simulink library "did"  (R2021b)
settings: Solver=VariableStepAuto  StartTime=0.0  StopTime=10.0  RelTol=1e-3
undefined symbols (not defined in the file or in its folder): ADID_DODRange_pct, ADID_SOCRange_pct, ADID_TempRange_C, DiscIntNeverNeededParam, ENUM_CHRGPLUGSTA_AC, ENUM_CHRGPLUGSTA_DC, ENUM_CHRGPLUGSTA_NONE, ENUM_DRIVETRAIN_AWD, ENUM_DRIVETRAIN_FWD, ENUM_DRIVETRAIN_RWD, ENUM_EXTCHRGSTS_CHARGING, ENUM_OBCV2LSTA_WORKING, ENUM_PWRSTASW_READY, ENUM_VEHICLETYPE_D31HAWD, ENUM_VEHICLETYPE_D31HRWD, HOUR2SEC, HUNDRED, KDID_CPSAVehSpdThres_kph, KDID_DIDModelVersion_raw, KDID_DoDChrgCycle_s, KDID_FiveKmEquivEnergy_Wh, KDID_FlashInitDIDModelVersion_raw, KDID_IPSAVehSpdThres_kph, KDID_PropActiveTripThres_s, KDID_PSARResetThres_sec, KDID_RESSCNTSDODRNGAXIS_enum, KDID_RESSTIMESOCRNGAXIS_enum, KDID_RESSTTEMPRNGAXIS_enum, KDID_WarnUpPropActiveThres_s, KDID_WarnUpVehOperIdleThres_mph, KDID_WarnUpVehOperIdleThres_s, KDID_WarnUpVehOperThres_mph, KDID_WarnUpVehOperThres_s, KPH2MPH, KXX2XX, MINUSONE_FLOAT, ONE_FLOAT, ONE_INT, ONE_INT16, ONE_PERCENT, TRUE, UINT16_MAX, UINT32_MAX, XX2KXX, ZERO_FLOAT, ZERO_INT, ZERO_INT16, ZERO_INT32
libraries: hcu_lib x112, simulink x10, nmm x1
(part 1 of 4)
settings Model: Creator=FVT23010  LastModifiedBy=FVT23010

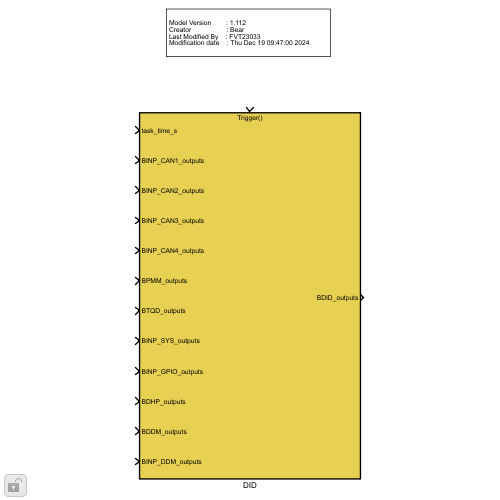
[thumbnail: Simulink's stored preview of the top-level diagram]
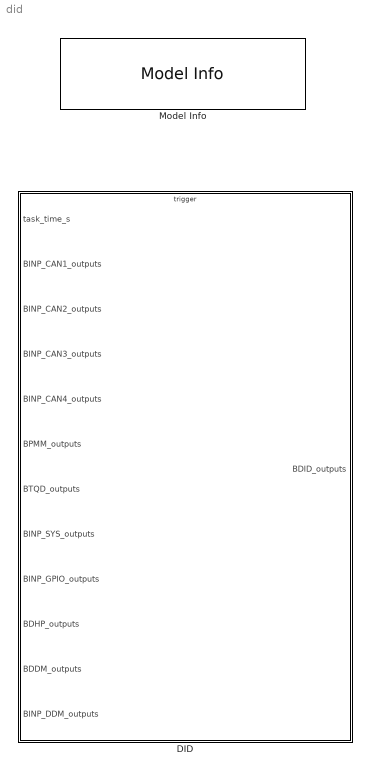
== system did ==
  DID : Subsystem
      settings: RTWSystemCode=Nonreusable function  RTWFcnNameOpts=Use subsystem name  RTWFileNameOpts=Use subsystem name
  Model Info : nmm/Model Info  InitialBlockCM=None  BlockCM=None  Frame=on  DisplayStringWithTags=|  HorizontalTextAlignment=Left  LeftAlignmentValue=0.02  SourceBlockDiagram=pmm  TagMaxNumber=20
      | Model Version        : %<ModelVersion>
      | Creator                   : Bear
      | Last Modified By    : %<LastModifiedBy>
      | Modification date    : %<LastModificationDate>

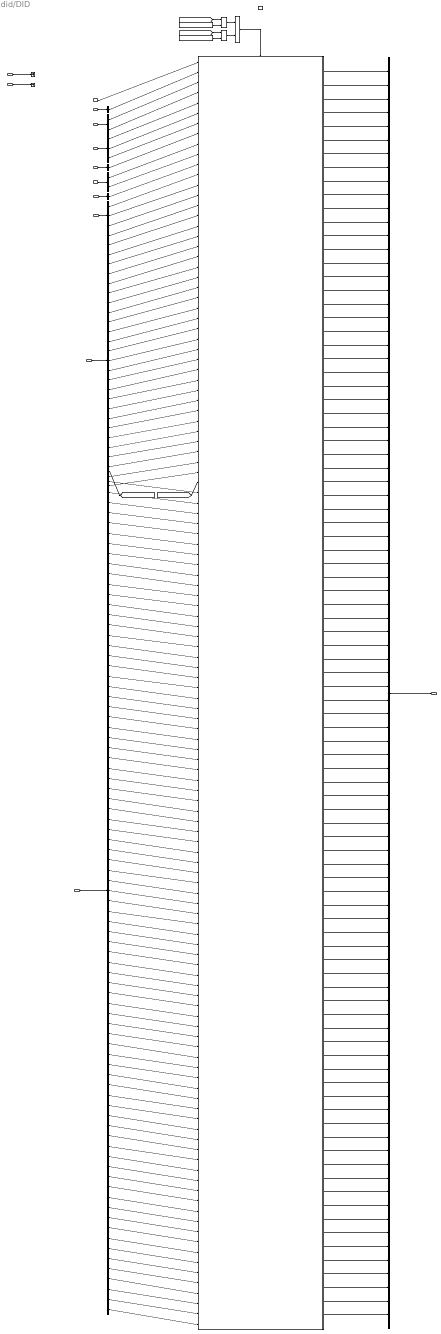
== system did/DID ==
  task_time_s : Inport
  BINP_CAN1_outputs : Inport  Port=2  OutDataTypeStr=Bus: BINP_CAN1_outputs
  BINP_CAN2_outputs : Inport  Port=3  OutDataTypeStr=Bus: BINP_CAN2_outputs
  BINP_CAN3_outputs : Inport  Port=4  OutDataTypeStr=Bus: BINP_CAN3_outputs
  BINP_CAN4_outputs : Inport  Port=5  OutDataTypeStr=Bus: BINP_CAN4_outputs
  BPMM_outputs : Inport  Port=6  OutDataTypeStr=Bus: BPMM_outputs
  BTQD_outputs : Inport  Port=7  OutDataTypeStr=Bus: BTQD_outputs
  BINP_SYS_outputs : Inport  Port=8  OutDataTypeStr=Bus: BINP_SYS_outputs
  BINP_GPIO_outputs : Inport  Port=9  OutDataTypeStr=Bus: BINP_GPIO_outputs
  BDHP_outputs : Inport  Port=10  OutDataTypeStr=Bus: BDHP_outputs
  BDDM_outputs : Inport  Port=11  OutDataTypeStr=Bus: BDDM_outputs
  BINP_DDM_outputs : Inport  Port=12  OutDataTypeStr=Bus: BINP_DDM_outputs
  Trigger : TriggerPort  TriggerType=function-call  VariantControl=(inherit)  PortDimensions=1
  Bus Creator : BusCreator  Inputs=92  OutDataTypeStr=Bus: BDID_outputs  NonVirtualBus=on
  Bus Selector : BusSelector  OutputSignals=VINP_VehicleType_enum,VINP_CarModel1_cnt,VINP_CarModel2_cnt,VINP_CarModel3_cnt,VINP_ECU1_cnt,VINP_ECU2_cnt,VINP_Major1_cnt,VINP_Major2_cnt,VINP_Minor1_cnt,VINP_Minor2_cnt,VINP_Patch1_cnt,VINP_Patch2_cnt,VINP_Country1_cnt,VINP_Country2_cnt,VINP_Variation_cnt,VINP_ECUGen1_cnt,VINP_ECUGen2_cnt,VINP_FlashMILDIST_km,VINP_FlashWARMUPS_cnt,VINP_FlashCLRDIST_km,VINP_FlashMILTIME_min,VINP_FlashCLRTIME_min,VINP_FlashNUMPSATRIPSFLTMEMCLR_cnt,VINP_FlashPSAR_sec,VINP_FlashPSAL_sec,VINP_FlashIPSAR_sec,VINP_FlashIPSAL_sec,VINP_FlashCPSAR_sec,VINP_FlashCPSAL_sec,VINP_FlashHVBNAH_Ahr,VINP_FlashIGNCNTR_cnt,VINP_FlashTNBCPSAR_Ahr,VINP_FlashTNBCPSAL_Ahr,VINP_FlashTNECPSAR_kWh,VINP_FlashTNECPSAL_kWh,VINP_FlashTEBPSAR_kWh,VINP_FlashTEBPSAL_kWh,VINP_FlashTGEOVCR_kWh,VINP_FlashTGEOVCL_kWh,VINP_FlashGECHGOVCDCR_kWh,VINP_FlashGECHGOVCDCL_kWh,VINP_FlashGECHGOVCACR_kWh,VINP_FlashGECHGOVCACL_kWh,VINP_FlashRESSV2XENNONPSAR_kWh,VINP_FlashRESSV2XENNONPSAL_kWh,VINP_FlashODOMETER_km,VINP_FlashPKERNumerator_kphsqr,VINP_FlashPKELNumerator_kphsqr,VINP_FlashResetCDEODTR_km,VINP_FlashBattTempPSAR_sec,VINP_FlashAvgBattTempPSAR_C,VINP_FlashBattTempPSAL_sec,VINP_FlashAvgBattTempPSAL_C,VINP_FlashOVCR_sec,VINP_FlashAvgBattTempOVCR_C,VINP_FlashOVCL_sec,VINP_FlashAvgBattTempOVCL_C,VINP_FlashOFFR_sec,VINP_FlashAvgBattTempOFFR_C,VINP_FlashOFFL_sec,VINP_FlashAvgBattTempOFFL_C,VINP_FlashHVBNE_kWh,VINP_FlashQTYPSATRIPSR_cnt,VINP_FlashQTYPSATRIPSL_cnt,VINP_FlashRESSCNTDODRNGR_cnt,VINP_FlashETMBTOER_kWh,VINP_FlashETMBTOEL_kWh,VINP_FlashRESSCNTDODRNGL_cnt,VINP_FlashETMATOER_kWh,VINP_FlashETMATOEL_kWh,VINP_FlashRESSTIMESOCPSARNGR_s,VINP_FlashRESSTIMESOCPSARNGL_s,VINP_FlashRESSTIMESOCCHGRNGR_s,VINP_FlashRESSTIMESOCOFFRNGL_s,VINP_FlashMAXBATTEMPL_C,VINP_FlashMINBATTEMPL_C,VINP_FlashRESSTIMESOCCHGRNGL_s,VINP_FlashRESSTIMESOCOFFRNGR_s,VINP_FlashAVGBATTEMPL_sec,VINP_FlashAVGBATTEMPL_C,VINP_VinCode_cnt,VINP_FlashDIDModelVersion_raw,VINP_FlashDIDModelVersionChkSum_raw
  Bus Selector1 : BusSelector  OutputSignals=VTQD_VehActSpd_kph
  Bus Selector2 : BusSelector  OutputSignals=VPMM_SysPowerMode_enum,VPMM_DrivetrainSelect_enum
  Bus Selector3 : BusSelector  OutputSignals=VDDM_VehMalfunLevel_enum,VDDM_LimpHomeActTmp_flg,VDDM_EnterNewOperCyc_flg
  Bus Selector4 : BusSelector  OutputSignals=VINP_ODOMETER_km,VINP_CANMsgValidMETER1_flg
  Bus Selector5 : BusSelector  OutputSignals=VINP_HVBattSOC_pct,VINP_HVBattPackVolt_V,VINP_ExtChrgSta_enum,VINP_HVBattCurr_A,VINP_HVBattVolt_V,VINP_ChrgPlugSta_enum,VINP_HVBPwrAvailChrg_kW,VINP_HVBCellVoltMax_mV,VINP_HVBCellVoltMin_mV,VINP_HVBSOH_pct,VINP_CANMsgValidMCUBR1_flg,VINP_CANMsgValidBMS6_flg,VINP_CANMsgValidBMS1_flg,VINP_CANMsgValidCCU2_flg,VINP_CANMsgValidBMS4_flg,VINP_CellTempAvg_C,VINP_OBCV2LSta_enum,VINP_RrMCUDCBusCurr_A,VINP_RrMCUDCBusVolt_V,VINP_FrMCUDCBusCurr_A,VINP_FrMCUDCBusVolt_V,VINP_CANMsgValidMCUBF1_flg,VINP_HVBMTempMax_C,VINP_HVBMTempMin_C,VINP_MCUBRRealPwrKwSta_kW,VINP_MCUBFRealPwrKwSta_kW,VINP_CANMsgValidBMS3_flg
  Bus Selector6 : BusSelector  OutputSignals=VINP_ClearDTCcmd_flg
  Bus Selector7 : BusSelector  OutputSignals=VDHP_LowIdleAccPedal_flg,VDHP_EAPS1NRM_pct,VDHP_EAPS2NRM_pct
  Bus Selector8 : BusSelector  OutputSignals=VINP_CANMsgValidESC1_flg
  Constant : Constant  Value=ENUM_VEHICLETYPE_D31HAWD
  Constant1 : Constant  Value=ENUM_VEHICLETYPE_D31HRWD
  Equal : RelationalOperator  Operator===  OutDataTypeStr=boolean  RndMeth=Simplest
  Equal1 : RelationalOperator  Operator===  OutDataTypeStr=boolean  RndMeth=Simplest
  Logical Operator : Logic  Operator=OR  AllPortsSameDT=off  OutDataTypeStr=boolean
  Subsystem : Subsystem
  Terminator : Terminator
  Terminator1 : Terminator
  BDID_outputs : Outport  OutDataTypeStr=Bus: BDID_outputs
  wires:
  BTQD_outputs/1 -> Bus Selector1/1
  task_time_s/1 -> Subsystem/1(task_time_s)
  Bus Selector1/1 -> Subsystem/2(VTQD_VehActSpd_kph)  "<VTQD_VehActSpd_kph>"
  BPMM_outputs/1 -> Bus Selector2/1
  Bus Selector2/1 -> Subsystem/3(VPMM_SysPowerMode_enum)  "<VPMM_SysPowerMode_enum>"
  BDDM_outputs/1 -> Bus Selector3/1
  BINP_CAN2_outputs/1 -> Bus Selector4/1
  Bus Selector3/1 -> Subsystem/5(VDDM_VehMalfunLevel_enum)  "<VDDM_VehMalfunLevel_enum>"
  Bus Selector4/1 -> Subsystem/9(VINP_ODOMETER_km)  "<VINP_ODOMETER_km>"
  BINP_DDM_outputs/1 -> Bus Selector6/1
  Bus Selector6/1 -> Subsystem/11(VINP_ClearDTCcmd_flg)  "<VINP_ClearDTCcmd_flg>"
  Bus Selector4/2 -> Subsystem/10(VINP_CANMsgValidMETER1_flg)  "<VINP_CANMsgValidMETER1_flg>"
  Bus Selector3/2 -> Subsystem/6(VDDM_LimpHomeActTmp_flg)  "<VDDM_LimpHomeActTmp_flg>"
  Bus Selector3/3 -> Subsystem/7(VDDM_EnterNewOperCyc_flg)  "<VDDM_EnterNewOperCyc_flg>"
  BDHP_outputs/1 -> Bus Selector7/1
  Bus Selector7/1 -> Subsystem/12(VDHP_LowIdleAccPedal_flg)  "<VDHP_LowIdleAccPedal_flg>"
  Bus Selector7/2 -> Subsystem/13(VDHP_EAPS1NRM_pct)  "<VDHP_EAPS1NRM_pct>"
  Bus Selector7/3 -> Subsystem/14(VDHP_EAPS2NRM_pct)  "<VDHP_EAPS2NRM_pct>"
  Bus Selector5/1 -> Subsystem/15(VINP_HVBattSOC_pct)  "<VINP_HVBattSOC_pct>"
  Bus Selector5/2 -> Subsystem/16(VINP_HVBattPackVolt_V)  "<VINP_HVBattPackVolt_V>"
  Constant/1 -> Equal/2
  Constant1/1 -> Equal1/2
  Equal/1 -> Logical Operator/1
  Equal1/1 -> Logical Operator/2
  Logical Operator/1 -> Subsystem/Enable
  Bus Selector5/3 -> Subsystem/17(VINP_ExtChrgSta_enum)  "<VINP_ExtChrgSta_enum>"
  BINP_CAN3_outputs/1 -> Bus Selector5/1
  Bus Selector5/4 -> Subsystem/18(VINP_HVBattCurr_A)  "<VINP_HVBattCurr_A>"
  Bus Selector5/5 -> Subsystem/19(VINP_HVBattVolt_V)  "<VINP_HVBattVolt_V>"
  Bus Selector5/6 -> Subsystem/20(VINP_ChrgPlugSta_enum)  "<VINP_ChrgPlugSta_enum>"
  Bus Selector5/7 -> Subsystem/21(VINP_HVBPwrAvailChrg_kW)  "<VINP_HVBPwrAvailChrg_kW>"
  Bus Selector5/8 -> Subsystem/22(VINP_HVBCellVoltMax_mV)  "<VINP_HVBCellVoltMax_mV>"
  Bus Selector5/9 -> Subsystem/23(VINP_HVBCellVoltMin_mV)  "<VINP_HVBCellVoltMin_mV>"
  Bus Selector5/10 -> Subsystem/24(VINP_HVBSOH_pct)  "<VINP_HVBSOH_pct>"
  BINP_CAN1_outputs/1 -> Bus Selector8/1  "BINP_CAN1_outputs"
  Bus Selector5/11 -> Subsystem/25(VINP_CANMsgValidMCUBR1_flg)  "<VINP_CANMsgValidMCUBR1_flg>"
  Bus Selector8/1 -> Subsystem/8(VINP_CANMsgValidESC1_flg)  "<VINP_CANMsgValidESC1_flg>"
  BINP_CAN4_outputs/1 -> Terminator/1
  BINP_GPIO_outputs/1 -> Terminator1/1
  Subsystem/4(VDID_WARMUPS_cnt) -> Bus Creator/4
  Subsystem/5(VDID_CLRDIST_km) -> Bus Creator/5
  Subsystem/3(VDID_MILDIST_km) -> Bus Creator/3
  Subsystem/6(VDID_APPD_pct) -> Bus Creator/6
  Subsystem/2(VDID_RUNTM_s) -> Bus Creator/2
  Subsystem/7(VDID_APPE_pct) -> Bus Creator/7
  Subsystem/1(VDID_VSS_kph) -> Bus Creator/1
  Subsystem/8(VDID_MILTIME_min) -> Bus Creator/8
  Subsystem/9(VDID_CLRTIME_min) -> Bus Creator/9
  Subsystem/10(VDID_BATSOC_pct) -> Bus Creator/10
  Subsystem/11(VDID_HEVBATT_V) -> Bus Creator/11
  Subsystem/12(VDID_ODOMETER_km) -> Bus Creator/12
  Subsystem/13(VDID_BATSOH_pct) -> Bus Creator/13
  Subsystem/14(VDID_HVBCellVoltMin_V) -> Bus Creator/14
  Subsystem/15(VDID_HVBCellVoltMax_V) -> Bus Creator/15
  Subsystem/16(VDID_HVESSCHARGELIM_kW) -> Bus Creator/16
  Subsystem/17(VDID_HVESSCHARGEACT_kW) -> Bus Creator/17
  Subsystem/18(VDID_HVESSENER_Whps) -> Bus Creator/18
  Subsystem/19(VDID_NUMPSATRIPSFLTMEMCLR_cnt) -> Bus Creator/19
  Subsystem/20(VDID_HVBattCurr_Ahps) -> Bus Creator/20
  Subsystem/21(VDID_PSAR_sec) -> Bus Creator/21
  Subsystem/22(VDID_PSAL_sec) -> Bus Creator/22
  Subsystem/23(VDID_IPSAR_sec) -> Bus Creator/23
  Subsystem/24(VDID_IPSAL_sec) -> Bus Creator/24
  Subsystem/25(VDID_CPSAR_sec) -> Bus Creator/25
  Subsystem/26(VDID_CPSAL_sec) -> Bus Creator/26
  Subsystem/27(VDID_HVBNAH_Ahr) -> Bus Creator/27
  Subsystem/28(VDID_HVBNE_kWh) -> Bus Creator/28
  Subsystem/29(VDID_IGNCNTR_cnt) -> Bus Creator/29
  Subsystem/30(VDID_TNBCPSAR_Ahr) -> Bus Creator/30
  Subsystem/31(VDID_TNBCPSAL_Ahr) -> Bus Creator/31
  Subsystem/32(VDID_TNECPSAR_kWh) -> Bus Creator/32
  Subsystem/33(VDID_TNECPSAL_kWh) -> Bus Creator/33
  Subsystem/34(VDID_TEBPSAR_kWh) -> Bus Creator/34
  Subsystem/35(VDID_TEBPSAL_kWh) -> Bus Creator/35
  Subsystem/36(VDID_TGEOVCR_kWh) -> Bus Creator/36
  Subsystem/37(VDID_TGEOVCL_kWh) -> Bus Creator/37
  Subsystem/38(VDID_GECHGOVCDCR_kWh) -> Bus Creator/38
  Subsystem/39(VDID_GECHGOVCDCL_kWh) -> Bus Creator/39
  Subsystem/40(VDID_GECHGOVCACR_kWh) -> Bus Creator/40
  Subsystem/41(VDID_GECHGOVCACL_kWh) -> Bus Creator/41
  Subsystem/42(VDID_RESSV2XENNONPSAR_kWh) -> Bus Creator/42
  Subsystem/43(VDID_RESSV2XENNONPSAL_kWh) -> Bus Creator/43
  Subsystem/44(VDID_PKER_kphsqr) -> Bus Creator/44
  Subsystem/45(VDID_PKEL_kphsqr) -> Bus Creator/45
  Subsystem/46(VDID_ResetCDEODTR_km) -> Bus Creator/46
  Subsystem/47(VDID_CDEODTR_km) -> Bus Creator/47
  Subsystem/48(VDID_CDEODTL_km) -> Bus Creator/48
  Subsystem/49(VDID_AvgBattTempPSAR_C) -> Bus Creator/49
  Subsystem/50(VDID_AvgBattTempPSAL_C) -> Bus Creator/50
  Subsystem/51(VDID_AvgBattTempOVCR_C) -> Bus Creator/51
  Subsystem/52(VDID_AvgBattTempOVCL_C) -> Bus Creator/52
  Subsystem/53(VDID_AvgBattTempOFFR_C) -> Bus Creator/53
  Subsystem/54(VDID_AvgBattTempOFFL_C) -> Bus Creator/54
  Bus Creator/1 -> BDID_outputs/1
  Bus Selector5/12 -> Subsystem/26(VINP_CANMsgValidBMS6_flg)  "<VINP_CANMsgValidBMS6_flg>"
  Bus Selector5/13 -> Subsystem/27(VINP_CANMsgValidBMS1_flg)  "<VINP_CANMsgValidBMS1_flg>"
  Bus Selector5/14 -> Subsystem/28(VINP_CANMsgValidCCU2_flg)  "<VINP_CANMsgValidCCU2_flg>"
  Bus Selector5/15 -> Subsystem/29(VINP_CANMsgValidBMS4_flg)  "<VINP_CANMsgValidBMS4_flg>"
  Bus Selector5/16 -> Subsystem/30(VINP_CellTempAvg_C)  "<VINP_CellTempAvg_C>"
  Bus Selector5/17 -> Subsystem/31(VINP_OBCV2LSta_enum)  "<VINP_OBCV2LSta_enum>"
  Subsystem/55(VDID_QTYPSATRIPSR_cnt) -> Bus Creator/55
  Subsystem/56(VDID_QTYPSATRIPSL_cnt) -> Bus Creator/56
  Subsystem/57(VDID_RESSCNTDODRNGR_cnt) -> Bus Creator/57
  Subsystem/58(VDID_RESSCNTDODRNGL_cnt) -> Bus Creator/58
  Subsystem/59(VDID_ETMATOER_kWh) -> Bus Creator/59
  Subsystem/60(VDID_ETMATOEL_kWh) -> Bus Creator/60
  Subsystem/61(VDID_ETMBTOER_kWh) -> Bus Creator/61
  Subsystem/62(VDID_ETMBTOEL_kWh) -> Bus Creator/62
  Subsystem/63(VDID_RESSTIMESOCPSARNGR_s) -> Bus Creator/63
  Subsystem/64(VDID_RESSTIMESOCPSARNGL_s) -> Bus Creator/64
  Subsystem/65(VDID_RESSTIMESOCCHGRNGR_s) -> Bus Creator/65
  Subsystem/66(VDID_RESSTIMESOCCHGRNGL_s) -> Bus Creator/66
  Subsystem/67(VDID_RESSTIMESOCOFFRNGR_s) -> Bus Creator/67
  Subsystem/68(VDID_RESSTIMESOCOFFRNGL_s) -> Bus Creator/68
  Subsystem/69(VDID_MAXBATTEMPL_C) -> Bus Creator/69
  Subsystem/70(VDID_MINBATTEMPL_C) -> Bus Creator/70
  Subsystem/71(VDID_AVGBATTEMPL_C) -> Bus Creator/71
  Subsystem/72(VDID_PRO TOCOLID_enum) -> Bus Creator/72
  Bus Selector5/24 -> Subsystem/38(VINP_HVBMTempMin_C)  "<VINP_HVBMTempMin_C>"
  Bus Selector5/23 -> Subsystem/37(VINP_HVBMTempMax_C)  "<VINP_HVBMTempMax_C>"
  Bus Selector5/22 -> Subsystem/36(VINP_CANMsgValidMCUBF1_flg)  "<VINP_CANMsgValidMCUBF1_flg>"
  Bus Selector5/21 -> Subsystem/35(VINP_FrMCUDCBusVolt_V)  "<VINP_FrMCUDCBusVolt_V>"
  Bus Selector5/20 -> Subsystem/34(VINP_FrMCUDCBusCurr_A)  "<VINP_FrMCUDCBusCurr_A>"
  Bus Selector5/19 -> Subsystem/33(VINP_RrMCUDCBusVolt_V)  "<VINP_RrMCUDCBusVolt_V>"
  Bus Selector5/18 -> Subsystem/32(VINP_RrMCUDCBusCurr_A)  "<VINP_RrMCUDCBusCurr_A>"
  Subsystem/73(VDID_RESSTTEMPRNGAXIS_enum) -> Bus Creator/73
  Subsystem/74(VDID_RESSTIMESOCRNGAXIS_enum) -> Bus Creator/74
  Subsystem/75(VDID_RESSCNTSDODRNGAXIS_enum) -> Bus Creator/75
  Bus Selector5/27 -> Subsystem/41(VINP_CANMsgValidBMS3_flg)  "<VINP_CANMsgValidBMS3_flg>"
  Bus Selector/2 -> Subsystem/43(VINP_CarModel1_cnt)  "<VINP_CarModel1_cnt>"
  Bus Selector/3 -> Subsystem/44(VINP_CarModel2_cnt)  "<VINP_CarModel2_cnt>"
  Bus Selector/4 -> Subsystem/45(VINP_CarModel3_cnt)  "<VINP_CarModel3_cnt>"
  Bus Selector/5 -> Subsystem/46(VINP_ECU1_cnt)  "<VINP_ECU1_cnt>"
  Bus Selector/6 -> Subsystem/47(VINP_ECU2_cnt)  "<VINP_ECU2_cnt>"
  Bus Selector/7 -> Subsystem/48(VINP_Major1_cnt)  "<VINP_Major1_cnt>"
  Bus Selector/8 -> Subsystem/49(VINP_Major2_cnt)  "<VINP_Major2_cnt>"
  Bus Selector/9 -> Subsystem/50(VINP_Minor1_cnt)  "<VINP_Minor1_cnt>"
  Bus Selector/10 -> Subsystem/51(VINP_Minor2_cnt)  "<VINP_Minor2_cnt>"
  Bus Selector/11 -> Subsystem/52(VINP_Patch1_cnt)  "<VINP_Patch1_cnt>"
  Bus Selector/12 -> Subsystem/53(VINP_Patch2_cnt)  "<VINP_Patch2_cnt>"
  Bus Selector/13 -> Subsystem/54(VINP_Country1_cnt)  "<VINP_Country1_cnt>"
  Bus Selector/14 -> Subsystem/55(VINP_Country2_cnt)  "<VINP_Country2_cnt>"
  Bus Selector/15 -> Subsystem/56(VINP_Variation_cnt)  "<VINP_Variation_cnt>"
  Bus Selector/16 -> Subsystem/57(VINP_ECUGen1_cnt)  "<VINP_ECUGen1_cnt>"
  Bus Selector/17 -> Subsystem/58(VINP_ECUGen2_cnt)  "<VINP_ECUGen2_cnt>"
  [VINP_VehicleType_enum] -> Equal/1
  [VINP_VehicleType_enum] -> Equal1/1
  Subsystem/76(VDID_CALID_cnt) -> Bus Creator/76
  Subsystem/77(VDID_ECUNAME_cnt) -> Bus Creator/77
  Subsystem/78(VDID_PKERNumerator_kphsqr) -> Bus Creator/78
  Subsystem/79(VDID_PKELNumerator_kphsqr) -> Bus Creator/79
  Subsystem/80(VDID_BattTempPSAR_sec) -> Bus Creator/80
  Subsystem/81(VDID_BattTempPSAL_sec) -> Bus Creator/81
  Subsystem/82(VDID_OVCR_sec) -> Bus Creator/82
  Subsystem/83(VDID_OVCL_sec) -> Bus Creator/83
  Subsystem/84(VDID_OFFR_sec) -> Bus Creator/84
  Subsystem/85(VDID_OFFL_sec) -> Bus Creator/85
  Subsystem/86(VDID_AVGBATTEMPL_sec) -> Bus Creator/86
  Bus Selector2/2 -> Subsystem/4(VPMM_DrivetrainSelect_enum)  "<VPMM_DrivetrainSelect_enum>"
  Bus Selector/18 -> Subsystem/59(VINP_FlashMILDIST_km)  "<VINP_FlashMILDIST_km>"
  Bus Selector/19 -> Subsystem/60(VINP_FlashWARMUPS_cnt)  "<VINP_FlashWARMUPS_cnt>"
  Bus Selector/20 -> Subsystem/61(VINP_FlashDelayCLRDIST_km)  "<VINP_FlashCLRDIST_km>"
  Bus Selector/21 -> Subsystem/62(VINP_FlashMILTime_min)  "<VINP_FlashMILTIME_min>"
  Bus Selector/22 -> Subsystem/63(VINP_FlashCLRTime_min)  "<VINP_FlashCLRTIME_min>"
  Bus Selector/23 -> Subsystem/64(VINP_FlashNUMPSATRIPSFLTMEMCLR_cnt)  "<VINP_FlashNUMPSATRIPSFLTMEMCLR_cnt>"
  Bus Selector/24 -> Subsystem/65(VINP_FlashPSAR_sec)  "<VINP_FlashPSAR_sec>"
  Bus Selector/25 -> Subsystem/66(VINP_FlashPSAL_sec)  "<VINP_FlashPSAL_sec>"
  Bus Selector/26 -> Subsystem/67(VINP_FlashIPSAR_sec)  "<VINP_FlashIPSAR_sec>"
  Bus Selector/27 -> Subsystem/68(VINP_FlashIPSAL_sec)  "<VINP_FlashIPSAL_sec>"
  Bus Selector/28 -> Subsystem/69(VINP_FlashCPSAR_sec)  "<VINP_FlashCPSAR_sec>"
  Bus Selector/29 -> Subsystem/70(VINP_FlashCPSAL_sec)  "<VINP_FlashCPSAL_sec>"
  Bus Selector/30 -> Subsystem/71(VINP_FlashHVBNAH_Ah)  "<VINP_FlashHVBNAH_Ahr>"
  Bus Selector/31 -> Subsystem/72(VINP_FlashIGNCNTR_cnt)  "<VINP_FlashIGNCNTR_cnt>"
  Bus Selector/32 -> Subsystem/73(VINP_FlashTNBCPSAR_Ahr)  "<VINP_FlashTNBCPSAR_Ahr>"
  Bus Selector/33 -> Subsystem/74(VINP_FlashTNBCPSAL_Ahr)  "<VINP_FlashTNBCPSAL_Ahr>"
  Bus Selector/34 -> Subsystem/75(VINP_FlashTNECPSAR_kWh)  "<VINP_FlashTNECPSAR_kWh>"
  Bus Selector/35 -> Subsystem/76(VINP_FlashTNECPSAL_kWh)  "<VINP_FlashTNECPSAL_kWh>"
  Bus Selector/36 -> Subsystem/77(VINP_FlashTEBPSAR_kWh)  "<VINP_FlashTEBPSAR_kWh>"
  Bus Selector/37 -> Subsystem/78(VINP_FlashTEBPSAL_kWh)  "<VINP_FlashTEBPSAL_kWh>"
  Bus Selector/38 -> Subsystem/79(VINP_FlashTGEOVCR_kWh)  "<VINP_FlashTGEOVCR_kWh>"
  Bus Selector/39 -> Subsystem/80(VINP_FlashTGEOVCL_kWh)  "<VINP_FlashTGEOVCL_kWh>"
  Bus Selector/40 -> Subsystem/81(VINP_FlashGECHGOVCDCR_kWh)  "<VINP_FlashGECHGOVCDCR_kWh>"
  Bus Selector/41 -> Subsystem/82(VINP_FlashGECHGOVCDCL_kWh)  "<VINP_FlashGECHGOVCDCL_kWh>"
  Bus Selector/42 -> Subsystem/83(VINP_FlashGECHGOVCACR_kWh)  "<VINP_FlashGECHGOVCACR_kWh>"
  Bus Selector/43 -> Subsystem/84(VINP_FlashGECHGOVCACL_kWh)  "<VINP_FlashGECHGOVCACL_kWh>"
  Bus Selector/44 -> Subsystem/85(VINP_FlashRESSV2XENNONPSAR_kWh)  "<VINP_FlashRESSV2XENNONPSAR_kWh>"
  Bus Selector/45 -> Subsystem/86(VINP_FlashRESSV2XENNONPSAL_kWh)  "<VINP_FlashRESSV2XENNONPSAL_kWh>"
  Bus Selector/46 -> Subsystem/87(VINP_FlashODOMETER_km)  "<VINP_FlashODOMETER_km>"
  Bus Selector/47 -> Subsystem/88(VINP_FlashPKERNumerator_kphsqr)  "<VINP_FlashPKERNumerator_kphsqr>"
  Bus Selector/48 -> Subsystem/89(VINP_FlashPKELNumerator_kphsqr)  "<VINP_FlashPKELNumerator_kphsqr>"
  Bus Selector/49 -> Subsystem/90(VINP_FlashResetCDEODTR_km)  "<VINP_FlashResetCDEODTR_km>"
  Bus Selector/50 -> Subsystem/91(VINP_FlashTempPSAR_sec)  "<VINP_FlashBattTempPSAR_sec>"
  Bus Selector/51 -> Subsystem/92(VINP_FlashAvgBattTempPSAR_C)  "<VINP_FlashAvgBattTempPSAR_C>"
  Bus Selector/52 -> Subsystem/93(VINP_FlashTempPSAL_sec)  "<VINP_FlashBattTempPSAL_sec>"
  Bus Selector/53 -> Subsystem/94(VINP_FlashAvgBattTempPSAL_C)  "<VINP_FlashAvgBattTempPSAL_C>"
  Bus Selector/54 -> Subsystem/95(VINP_FlashOVCR_sec)  "<VINP_FlashOVCR_sec>"
  Bus Selector/55 -> Subsystem/96(VINP_FlashAvgBattTempOVCR_C)  "<VINP_FlashAvgBattTempOVCR_C>"
  Bus Selector/56 -> Subsystem/97(VINP_FlashOVCL_sec)  "<VINP_FlashOVCL_sec>"
  Bus Selector/57 -> Subsystem/98(VINP_FlashAvgBattTempOVCL_C)  "<VINP_FlashAvgBattTempOVCL_C>"
  Bus Selector/58 -> Subsystem/99(VINP_FlashOFFR_sec)  "<VINP_FlashOFFR_sec>"
  Bus Selector/59 -> Subsystem/100(VINP_FlashAvgBattTempOFFR_C)  "<VINP_FlashAvgBattTempOFFR_C>"
  Bus Selector/60 -> Subsystem/101(VINP_FlashOFFL_sec)  "<VINP_FlashOFFL_sec>"
  Bus Selector/61 -> Subsystem/102(VINP_FlashAvgBattTempOFFL_C)  "<VINP_FlashAvgBattTempOFFL_C>"
  Bus Selector/62 -> Subsystem/103(VINP_FlashHVBNE_kWh)  "<VINP_FlashHVBNE_kWh>"
  Bus Selector/63 -> Subsystem/104(VINP_FlashQTYPSATRIPSR_cnt)  "<VINP_FlashQTYPSATRIPSR_cnt>"
  Bus Selector/64 -> Subsystem/105(VINP_FlashQTYPSATRIPSL_cnt)  "<VINP_FlashQTYPSATRIPSL_cnt>"
  Bus Selector/65 -> Subsystem/106(VINP_FlashRESSCNTDODRNGR_cnt)  "<VINP_FlashRESSCNTDODRNGR_cnt>"
  Bus Selector/71 -> Subsystem/112(VINP_FlashRESSTIMESOCPSARNGR_s)  "<VINP_FlashRESSTIMESOCPSARNGR_s>"
  Bus Selector/72 -> Subsystem/113(VINP_FlashRESSTIMESOCPSARNGL_s)  "<VINP_FlashRESSTIMESOCPSARNGL_s>"
  Bus Selector/73 -> Subsystem/114(VINP_FlashRESSTIMESOCCHGRNGR_s)  "<VINP_FlashRESSTIMESOCCHGRNGR_s>"
  Bus Selector/79 -> Subsystem/120(VINP_FlashAVGBATTEMPL_sec)  "<VINP_FlashAVGBATTEMPL_sec>"
  Bus Selector/80 -> Subsystem/121(VINP_FlashAVGBATTEMPL_C)  "<VINP_FlashAVGBATTEMPL_C>"
  Bus Selector/78 -> Subsystem/119(VINP_FlashRESSTIMESOCOFFRNGR_s)  "<VINP_FlashRESSTIMESOCOFFRNGR_s>"
  Bus Selector/74 -> Subsystem/115(VINP_FlashRESSTIMESOCOFFRNGL_s)  "<VINP_FlashRESSTIMESOCOFFRNGL_s>"
  Bus Selector/75 -> Subsystem/116(VINP_FlashMAXBATTEMPL_C)  "<VINP_FlashMAXBATTEMPL_C>"
  Bus Selector/76 -> Subsystem/117(VINP_FlashMINBATTEMPL_C)  "<VINP_FlashMINBATTEMPL_C>"
  Bus Selector/77 -> Subsystem/118(VINP_FlashRESSTIMESOCCHGRNGL_s)  "<VINP_FlashRESSTIMESOCCHGRNGL_s>"
  Bus Selector/66 -> Subsystem/107(VINP_FlashETMBTOER_kWh)  "<VINP_FlashETMBTOER_kWh>"
  Bus Selector/67 -> Subsystem/108(VINP_FlashETMBTOEL_kWh)  "<VINP_FlashETMBTOEL_kWh>"
  Bus Selector/68 -> Subsystem/109(VINP_FlashRESSCNTDODRNGL_cnt)  "<VINP_FlashRESSCNTDODRNGL_cnt>"
  Bus Selector/69 -> Subsystem/110(VINP_FlashETMATOER_kWh)  "<VINP_FlashETMATOER_kWh>"
  Bus Selector/70 -> Subsystem/111(VINP_FlashETMATOEL_kWh)  "<VINP_FlashETMATOEL_kWh>"
  Bus Selector/81 -> Subsystem/122(VINP_VinCode_cnt)  "<VINP_VinCode_cnt>"
  BINP_SYS_outputs/1 -> Bus Selector/1
  Bus Selector/1 -> [VINP_VehicleType_enum]  "<VINP_VehicleType_enum>"
  [VINP_VehicleType_enum] -> Subsystem/42(VINP_VehicleType_enum)
  Bus Selector5/25 -> Subsystem/39(VINP_MCUBRRealPwrKwSta_kW)  "<VINP_MCUBRRealPwrKwSta_kW>"
  Bus Selector5/26 -> Subsystem/40(VINP_MCUBFRealPwrKwSta_kW)  "<VINP_MCUBFRealPwrKwSta_kW>"
  Subsystem/87(VDID_VinCode_cnt) -> Bus Creator/87
  Subsystem/88(VDID_STASUP_enum) -> Bus Creator/88
  Subsystem/89(VDID_HEVMODE_enum) -> Bus Creator/89
  Subsystem/90(VDID_HVBATT_A) -> Bus Creator/90
  Subsystem/91(VDID_DIDModelVersion_raw) -> Bus Creator/91
  Subsystem/92(VDID_DIDModelVersionChksum_raw) -> Bus Creator/92
  Bus Selector/82 -> Subsystem/123(VINP_FlashModelVersion_raw)  "<VINP_FlashDIDModelVersion_raw>"
  Bus Selector/83 -> Subsystem/124(VINP_FlashModelVersionChksum_raw)  "<VINP_FlashDIDModelVersionChkSum_raw>"
